simulink model "automaticWiperController"  (R2024b)
settings: Solver=VariableStepAuto  StartTime=0.0  StopTime=10.0  RelTol=1e-3
undefined symbols (not defined in the file or in its folder): intensityEnum, onOffEnum, wiperSpeedEnum
libraries: simulink x1
settings Model: Creator=ACER  LastModifiedBy=ACER

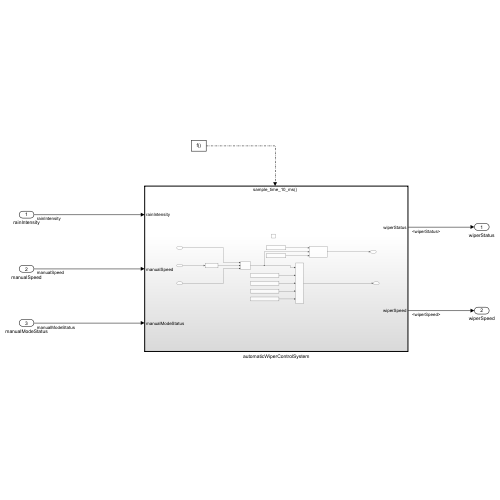
[thumbnail: Simulink's stored preview of the top-level diagram]
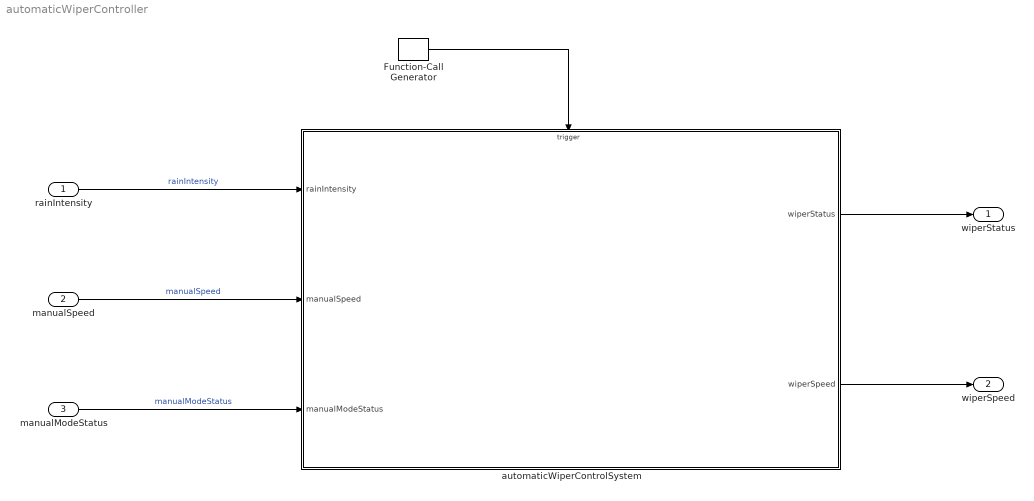
== system automaticWiperController ==
  rainIntensity : Inport  OutDataTypeStr=Enum: intensityEnum
  manualSpeed : Inport  Port=2  OutDataTypeStr=Enum: intensityEnum
  manualModeStatus : Inport  Port=3  OutDataTypeStr=Enum: onOffEnum
  Function-Call Generator : simulink/Ports & Subsystems/Function-Call Generator  sample_time=0.01  numberOfIterations=1  DisallowWideOutput=off
  automaticWiperControlSystem : Subsystem
  wiperStatus : Outport
  wiperSpeed : Outport  Port=2
  wires:
  Function-Call Generator/1 -> automaticWiperControlSystem/Trigger
  rainIntensity/1 -> automaticWiperControlSystem/1(rainIntensity)  "rainIntensity"
  manualSpeed/1 -> automaticWiperControlSystem/2(manualSpeed)  "manualSpeed"
  automaticWiperControlSystem/1(wiperStatus) -> wiperStatus/1
  automaticWiperControlSystem/2(wiperSpeed) -> wiperSpeed/1
  manualModeStatus/1 -> automaticWiperControlSystem/3(manualModeStatus)  "manualModeStatus"

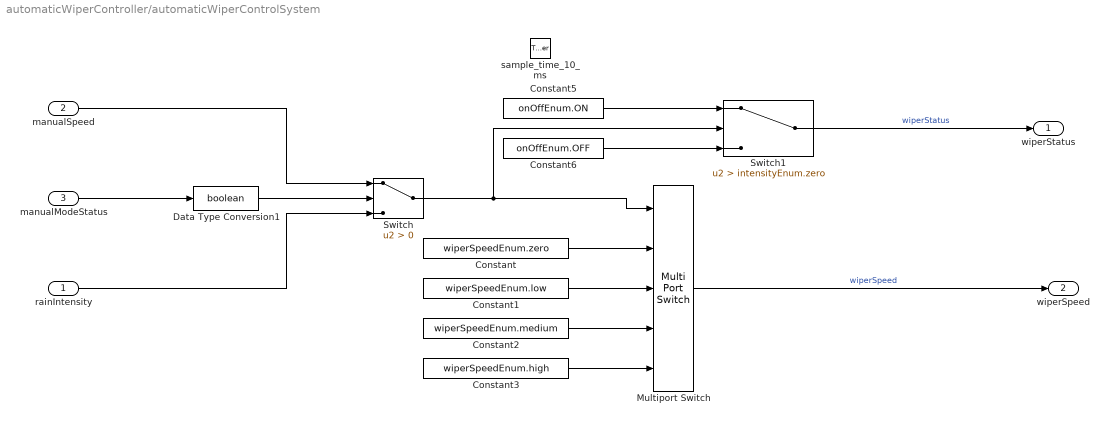
== system automaticWiperController/automaticWiperControlSystem ==
  rainIntensity : Inport
  manualSpeed : Inport  Port=2
  manualModeStatus : Inport  Port=3
  sample_time_10_ms : TriggerPort  TriggerType=function-call  VariantControl=(inherit)  SampleTimeType=periodic  SampleTime=0.01  PortDimensions=1
  Constant : Constant  Value=wiperSpeedEnum.zero
  Constant1 : Constant  Value=wiperSpeedEnum.low
  Constant2 : Constant  Value=wiperSpeedEnum.medium
  Constant3 : Constant  Value=wiperSpeedEnum.high
  Constant5 : Constant  Value=onOffEnum.ON
  Constant6 : Constant  Value=onOffEnum.OFF
  Data Type Conversion1 : DataTypeConversion  OutDataTypeStr=boolean  SaturateOnIntegerOverflow=off  RndMeth=Floor
  Multiport Switch : MultiPortSwitch  DataPortOrder=Specify indices  Inputs=4  DataPortIndices={intensityEnum.zero,intensityEnum.low,intensityEnum.medium,intensityEnum.high}  DiagnosticForDefault=None  SaturateOnIntegerOverflow=off  InputSameDT=off
  Switch : Switch  Criteria=u2 > Threshold  SaturateOnIntegerOverflow=off  InputSameDT=off
  Switch1 : Switch  Criteria=u2 > Threshold  Threshold=intensityEnum.zero  SaturateOnIntegerOverflow=off  InputSameDT=off
  wiperStatus : Outport  OutDataTypeStr=Enum: onOffEnum  InitialOutput=onOffEnum.OFF
  wiperSpeed : Outport  Port=2  OutDataTypeStr=Enum: wiperSpeedEnum  InitialOutput=wiperSpeedEnum.zero
  wires:
  Multiport Switch/1 -> wiperSpeed/1  "wiperSpeed"
  manualModeStatus/1 -> Data Type Conversion1/1
  rainIntensity/1 -> Switch/3
  Switch1/1 -> wiperStatus/1  "wiperStatus"
  Constant5/1 -> Switch1/1
  Constant6/1 -> Switch1/3
  Constant/1 -> Multiport Switch/2
  Constant1/1 -> Multiport Switch/3
  Constant2/1 -> Multiport Switch/4
  Constant3/1 -> Multiport Switch/5
  Switch/1 -> Multiport Switch/1, Switch1/2
  Data Type Conversion1/1 -> Switch/2
  manualSpeed/1 -> Switch/1
